simulink model "PMSMmathmodelling"  (R2020a)
settings: Solver=VariableStepAuto  StartTime=0.0  StopTime=10.0  RelTol=1e-3
values from neighbouring files (symbols this model uses):
  flux_m = 1    [constantsPMSM.m]
  flux_ref = 0    [constantsPMSM.m]
  K_icd = 1    [constantsPMSM.m]
  K_icq = 1    [constantsPMSM.m]
  K_pcd = K_p_d    (= 0.002728370453)    [constantsPMSM.m]
  K_pcq = K_p_q    (= 0.002728370453)    [constantsPMSM.m]
  kp_flux_gain = 1    [constantsPMSM.m]
  kp_speed_gain = 1    [constantsPMSM.m]
  w_r_ref = 10    [constantsPMSM.m]
  x_d = x_s_sigma + x_ad    (= 2)    [constantsPMSM.m]
  x_q = x_s_sigma + x_aq    (= 2)    [constantsPMSM.m]
libraries: mcbcontrolslib x4, simulink x2
settings Model: Creator=mahoyen  LastModifiedBy=mahoyen

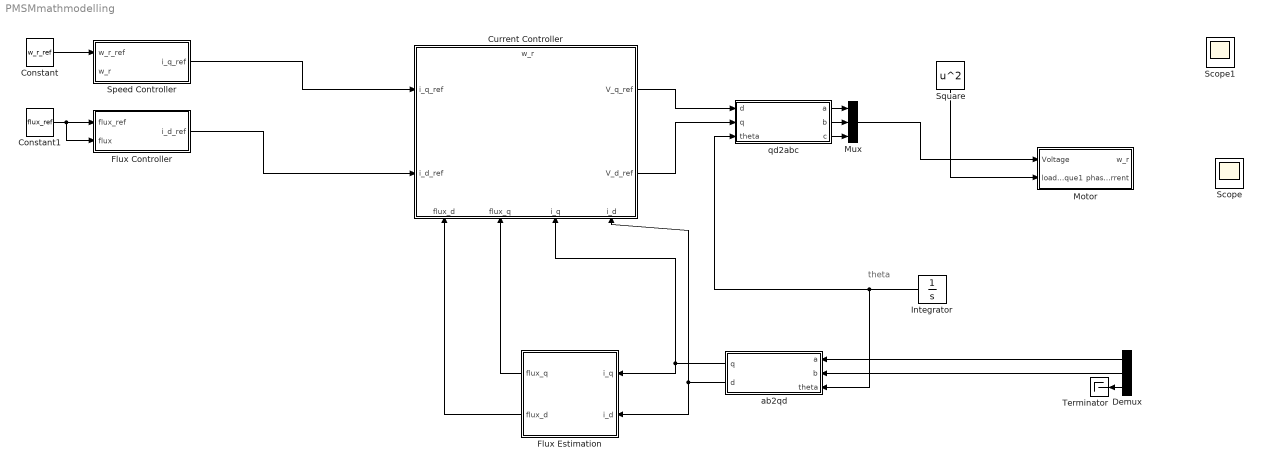
== system PMSMmathmodelling ==
  note: theta
  Constant : Constant  Value=w_r_ref
  Constant1 : Constant  Value=flux_ref
  Current Controller : Subsystem
      settings: PortSchema="{\"entries\":[{\"content\":{\"sides\":[{\"content\":{\"connectorIds\":[\"In1\",\"In2\"]},\"type\":\"ConnectorPlacement.EquallySpacedRectSide\",\"uuid\":\"d2db9237-7a25-4972-ad11-fca93cfe0796\"},{\"content\":{\"connectorIds\":[\"Out1\",\"Out2\"],\"side\":\"RIGHT\"},\"type\":\"ConnectorPlacement.EquallySpacedRectSide\",\"uuid\":\"de3236f9-3478-4b60-a0f6-95c46eb50464\"},{\"content\":{\"connectorIds\":[\"In3\"],\"side\":\"TOP\"},\"type\":\"ConnectorPlacement.EquallySpacedRectSide\",\"uuid\":\"449a4802-8b8b-4f05-8e5e-518b92a53f63\"},{\"content\":{\"connectorIds\":[\"In4\",\"In5\",\"In6\",\"In7\"],\"side\":\"BOTTOM\"},\"type\":\"ConnectorPlacement.EquallySpacedRectSide\",\"uuid\":\"10a1e68a-bb9c-4b2f-8ec0-0ff13f85575e\"}]},\"type\":\"ConnectorPlacement.EquallySpacedConnector\",\"uuid\":\"9560f9d1-6062-4328-885c-1a76f0563ab6\"}],\"packageUris\":[\"http://schema.mathworks.com/mf0/Connector/19700101\"],\"version\":\"1.0\"}"
  Demux : Demux  Outputs=3
  Flux Controller : Subsystem
  Flux Estimation : Subsystem
  Integrator : Integrator
  Motor : Subsystem
  Mux : Mux  Inputs=3
  Scope : Scope
  Scope1 : Scope
  Speed Controller : Subsystem
  Square : Math  Operator=square  SaturateOnIntegerOverflow=on
  Terminator : Terminator
  ab2qd : Subsystem
  qd2abc : Subsystem
  wires:
  Speed Controller/1(i_q_ref) -> Current Controller/1(i_q_ref)
  Flux Controller/1(i_d_ref) -> Current Controller/2(i_d_ref)
  qd2abc/1(a) -> Mux/1
  qd2abc/3(c) -> Mux/3
  qd2abc/2(b) -> Mux/2
  Mux/1 -> Motor/1(Voltage)
  Current Controller/1(V_q_ref) -> qd2abc/1(d)
  Current Controller/2(V_d_ref) -> qd2abc/2(q)
  ? -> Integrator/1, Scope1/1, Square/1, Speed Controller/2(w_r), Current Controller/3(w_r)
  Integrator/1 -> qd2abc/3(theta), ab2qd/3(theta)
  Square/1 -> Motor/2(load_torque1)
  ? -> Demux/1, Scope/1
  Demux/1 -> ab2qd/1(a)
  Demux/2 -> ab2qd/2(b)
  Demux/3 -> Terminator/1
  ab2qd/2(d) -> Flux Estimation/2(i_d), Current Controller/7(i_d)
  ab2qd/1(q) -> Current Controller/6(i_q), Flux Estimation/1(i_q)
  Flux Estimation/1(flux_q) -> Current Controller/5(flux_q)
  Flux Estimation/2(flux_d) -> Current Controller/4(flux_d)
  Constant/1 -> Speed Controller/1(w_r_ref)
  Constant1/1 -> Flux Controller/2(flux), Flux Controller/1(flux_ref)

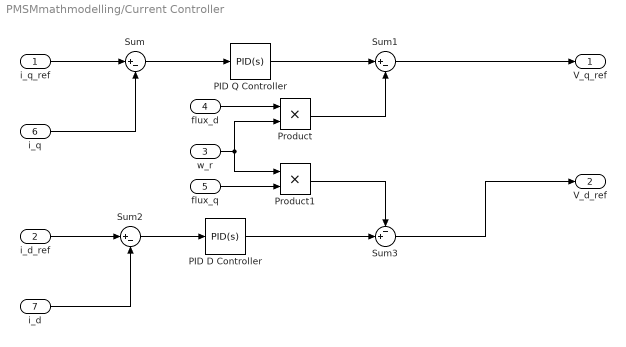
== system PMSMmathmodelling/Current Controller ==
  i_q_ref : Inport
  i_d_ref : Inport  Port=2
  w_r : Inport  Port=3
  flux_d : Inport  Port=4
  flux_q : Inport  Port=5
  i_q : Inport  Port=6
  i_d : Inport  Port=7
  PID D Controller : simulink/Continuous/PID Controller  Controller=PID  Form=Parallel  TimeDomain=Continuous-time  UseExternalTs=off  SampleTime=-1  IntegratorMethod=Forward Euler  FilterMethod=Forward Euler  ControllerParametersSource=internal  P=K_pcd  I=K_icd  D=0  UseFilter=on  N=100  TunerSelectOption=Transfer Function Based (PID Tuner App)  InitialConditionSource=internal  InitialConditionForIntegrator=0  InitialConditionForFilter=0  DifferentiatorICPrevScaledInput=0  ExternalReset=none  TrackingMode=off  Kt=1  LimitOutput=off  UpperSaturationLimit=inf  LowerSaturationLimit=-inf  LinearizeAsGain=on  AntiWindupMode=none  Kb=1  POutMin=[]  POutMax=[]  IOutMin=[]  IOutMax=[]  DOutMin=[]  DOutMax=[]  NOutMin=[]  NOutMax=[]  SumOutMin=[]  SumOutMax=[]  SaturationOutMin=[]  SaturationOutMax=[]  PParamMin=[]  PParamMax=[]  IParamMin=[]  IParamMax=[]  DParamMin=[]  DParamMax=[]  NParamMin=[]  NParamMax=[]  KbParamMin=[]  KbParamMax=[]  KtParamMin=[]  KtParamMax=[]  KbOutMin=[]  KbOutMax=[]  KtOutMin=[]  KtOutMax=[]  IntegratorOutMin=[]  IntegratorOutMax=[]  FilterOutMin=[]  FilterOutMax=[]  SumI1OutMin=[]  SumI1OutMax=[]  SumI2OutMin=[]  SumI2OutMax=[]  SumI3OutMin=[]  SumI3OutMax=[]  SumI4OutMin=[]  SumI4OutMax=[]  SumDOutMin=[]  SumDOutMax=[]  DifferentiatorOutMin=[]  DifferentiatorOutMax=[]  FilterDiffOutCoefMin=[]  FilterDiffOutCoefMax=[]  ReciprocalOutMin=[]  ReciprocalOutMax=[]  SumDenOutMin=[]  SumDenOutMax=[]  SumNumOutMin=[]  SumNumOutMax=[]  DivideOutMin=[]  DivideOutMax=[]  UdiffTsProdOutMin=[]  UdiffTsProdOutMax=[]  NTsProdOutMin=[]  NTsProdOutMax=[]  UintegralTsProdOutMin=[]  UintegralTsProdOutMax=[]  UngainTsProdOutMin=[]  UngainTsProdOutMax=[]  IntegratorContinuousStateAttributes=''  IntegratorStateMustResolveToSignalObject=off  IntegratorRTWStateStorageClass=Auto  FilterContinuousStateAttributes=''  FilterStateMustResolveToSignalObject=off  FilterRTWStateStorageClass=Auto  ParallelPVariant=InternalParameters  IdealPVariant=Disabled  IVariant=InternalParameters  DVariant=InternalParameters  IntegratorVariant=Continuous  SatVariant=Disabled  AWVariant=Passthrough  PCopyVariant=Disabled  TRVariant=Disabled  FdbkBlocksVariant=Forward  IdealPFdbkVariant=Disabled  SatFdbkVariant=Disabled  DerivativeFilterVariant=ContFilter  NVariant=InternalParameters  NCopyVariant=Disabled  FilterICVariant=InternalICsFilter  IntegratorICVariant=InternalICs  ExternalResetVariant=Disabled  TRSumVariant=Passthrough  SumFdbkVariant=Disabled  SumVariant=Sum_PID  TsampFilterVariant=InternalTs  TsampNgainVariant=Passthrough  TsampIntegralVariant=Passthrough
  PID Q Controller : simulink/Continuous/PID Controller  Controller=PID  Form=Parallel  TimeDomain=Continuous-time  UseExternalTs=off  SampleTime=-1  IntegratorMethod=Forward Euler  FilterMethod=Forward Euler  ControllerParametersSource=internal  P=K_pcq  I=K_icq  D=0  UseFilter=on  N=100  TunerSelectOption=Transfer Function Based (PID Tuner App)  InitialConditionSource=internal  InitialConditionForIntegrator=0  InitialConditionForFilter=0  DifferentiatorICPrevScaledInput=0  ExternalReset=none  TrackingMode=off  Kt=1  LimitOutput=off  UpperSaturationLimit=inf  LowerSaturationLimit=-inf  LinearizeAsGain=on  AntiWindupMode=none  Kb=1  POutMin=[]  POutMax=[]  IOutMin=[]  IOutMax=[]  DOutMin=[]  DOutMax=[]  NOutMin=[]  NOutMax=[]  SumOutMin=[]  SumOutMax=[]  SaturationOutMin=[]  SaturationOutMax=[]  PParamMin=[]  PParamMax=[]  IParamMin=[]  IParamMax=[]  DParamMin=[]  DParamMax=[]  NParamMin=[]  NParamMax=[]  KbParamMin=[]  KbParamMax=[]  KtParamMin=[]  KtParamMax=[]  KbOutMin=[]  KbOutMax=[]  KtOutMin=[]  KtOutMax=[]  IntegratorOutMin=[]  IntegratorOutMax=[]  FilterOutMin=[]  FilterOutMax=[]  SumI1OutMin=[]  SumI1OutMax=[]  SumI2OutMin=[]  SumI2OutMax=[]  SumI3OutMin=[]  SumI3OutMax=[]  SumI4OutMin=[]  SumI4OutMax=[]  SumDOutMin=[]  SumDOutMax=[]  DifferentiatorOutMin=[]  DifferentiatorOutMax=[]  FilterDiffOutCoefMin=[]  FilterDiffOutCoefMax=[]  ReciprocalOutMin=[]  ReciprocalOutMax=[]  SumDenOutMin=[]  SumDenOutMax=[]  SumNumOutMin=[]  SumNumOutMax=[]  DivideOutMin=[]  DivideOutMax=[]  UdiffTsProdOutMin=[]  UdiffTsProdOutMax=[]  NTsProdOutMin=[]  NTsProdOutMax=[]  UintegralTsProdOutMin=[]  UintegralTsProdOutMax=[]  UngainTsProdOutMin=[]  UngainTsProdOutMax=[]  IntegratorContinuousStateAttributes=''  IntegratorStateMustResolveToSignalObject=off  IntegratorRTWStateStorageClass=Auto  FilterContinuousStateAttributes=''  FilterStateMustResolveToSignalObject=off  FilterRTWStateStorageClass=Auto  ParallelPVariant=InternalParameters  IdealPVariant=Disabled  IVariant=InternalParameters  DVariant=InternalParameters  IntegratorVariant=Continuous  SatVariant=Disabled  AWVariant=Passthrough  PCopyVariant=Disabled  TRVariant=Disabled  FdbkBlocksVariant=Forward  IdealPFdbkVariant=Disabled  SatFdbkVariant=Disabled  DerivativeFilterVariant=ContFilter  NVariant=InternalParameters  NCopyVariant=Disabled  FilterICVariant=InternalICsFilter  IntegratorICVariant=InternalICs  ExternalResetVariant=Disabled  TRSumVariant=Passthrough  SumFdbkVariant=Disabled  SumVariant=Sum_PID  TsampFilterVariant=InternalTs  TsampNgainVariant=Passthrough  TsampIntegralVariant=Passthrough
  Product : Product
  Product1 : Product
  Sum : Sum  Inputs=|+-
  Sum1 : Sum  Inputs=|+-
  Sum2 : Sum  Inputs=|+-
  Sum3 : Sum  Inputs=-+|
  V_q_ref : Outport
  V_d_ref : Outport  Port=2
  wires:
  i_q_ref/1 -> Sum/1
  i_q/1 -> Sum/2
  Sum/1 -> PID Q Controller/1
  PID Q Controller/1 -> Sum1/1
  Product/1 -> Sum1/2
  Sum1/1 -> V_q_ref/1
  w_r/1 -> Product1/1, Product/2
  Sum3/1 -> V_d_ref/1
  i_d/1 -> Sum2/2
  Sum2/1 -> PID D Controller/1
  i_d_ref/1 -> Sum2/1
  Product1/1 -> Sum3/1
  PID D Controller/1 -> Sum3/2
  flux_d/1 -> Product/1
  flux_q/1 -> Product1/2

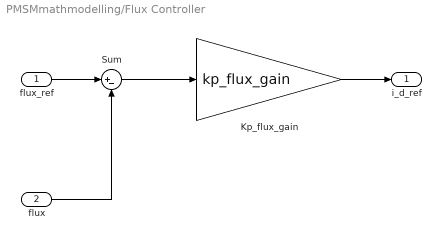
== system PMSMmathmodelling/Flux Controller ==
  flux_ref : Inport
  flux : Inport  Port=2
  Kp_flux_gain : Gain  Gain=kp_flux_gain
  Sum : Sum  Inputs=|+-
  i_d_ref : Outport
  wires:
  flux_ref/1 -> Sum/1
  flux/1 -> Sum/2
  Sum/1 -> Kp_flux_gain/1
  Kp_flux_gain/1 -> i_d_ref/1

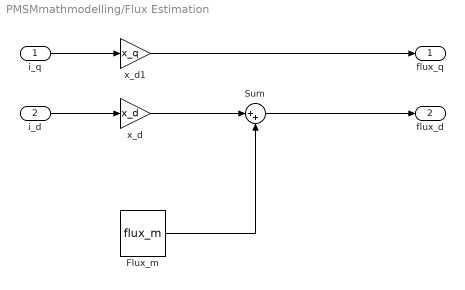
== system PMSMmathmodelling/Flux Estimation ==
  i_q : Inport
  i_d : Inport  Port=2
  Flux_m : Constant  Value=flux_m
  Sum : Sum  Inputs=|++
  x_d : Gain  Gain=x_d
  x_d1 : Gain  Gain=x_q
  flux_q : Outport
  flux_d : Outport  Port=2
  wires:
  i_d/1 -> x_d/1
  i_q/1 -> x_d1/1
  x_d/1 -> Sum/1
  Sum/1 -> flux_d/1
  Flux_m/1 -> Sum/2
  x_d1/1 -> flux_q/1

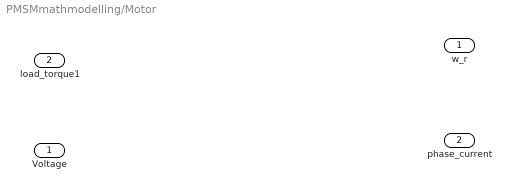
== system PMSMmathmodelling/Motor ==
  Voltage : Inport
  load_torque1 : Inport  Port=2
  w_r : Outport
  phase_current : Outport  Port=2

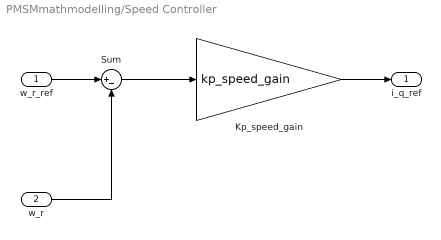
== system PMSMmathmodelling/Speed Controller ==
  w_r_ref : Inport
  w_r : Inport  Port=2
  Kp_speed_gain : Gain  Gain=kp_speed_gain
  Sum : Sum  Inputs=|+-
  i_q_ref : Outport
  wires:
  w_r_ref/1 -> Sum/1
  w_r/1 -> Sum/2
  Sum/1 -> Kp_speed_gain/1
  Kp_speed_gain/1 -> i_q_ref/1

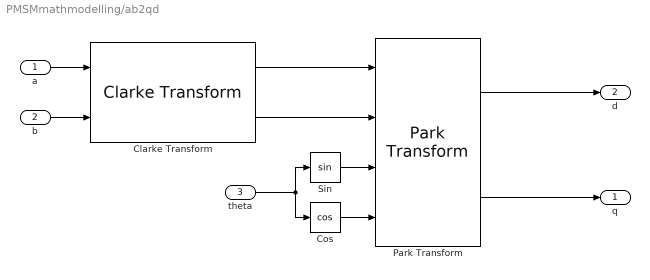
== system PMSMmathmodelling/ab2qd ==
  a : Inport
  b : Inport  Port=2
  theta : Inport  Port=3
  Clarke Transform : mcbcontrolslib/Clarke Transform  VariantControl=Variant2
  Cos : Trigonometry  Operator=cos
  Park Transform : mcbcontrolslib/Park Transform  AxisAlignment=D-axis
      settings: SourceProductBaseCode=MT
  Sin : Trigonometry
  q : Outport
  d : Outport  Port=2
  wires:
  a/1 -> Clarke Transform/1
  b/1 -> Clarke Transform/2
  theta/1 -> Cos/1, Sin/1
  Sin/1 -> Park Transform/3
  Cos/1 -> Park Transform/4
  Clarke Transform/1 -> Park Transform/1
  Clarke Transform/2 -> Park Transform/2
  Park Transform/2 -> q/1
  Park Transform/1 -> d/1

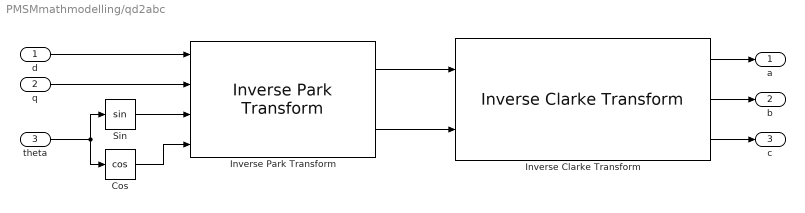
== system PMSMmathmodelling/qd2abc ==
  d : Inport
  q : Inport  Port=2
  theta : Inport  Port=3
  Cos : Trigonometry  Operator=cos
  Inverse Clarke Transform : mcbcontrolslib/Inverse Clarke Transform
      settings: SourceProductBaseCode=MT
  Inverse Park Transform : mcbcontrolslib/Inverse Park Transform  AxisAlignment=D-axis
  Sin : Trigonometry
  a : Outport
  b : Outport  Port=2
  c : Outport  Port=3
  wires:
  Inverse Park Transform/1 -> Inverse Clarke Transform/1
  Inverse Park Transform/2 -> Inverse Clarke Transform/2
  d/1 -> Inverse Park Transform/1
  q/1 -> Inverse Park Transform/2
  theta/1 -> Cos/1, Sin/1
  Sin/1 -> Inverse Park Transform/3
  Cos/1 -> Inverse Park Transform/4
  Inverse Clarke Transform/2 -> b/1
  Inverse Clarke Transform/3 -> c/1
  Inverse Clarke Transform/1 -> a/1
